simulink model "LocalPlannerMPCCascade"  (R2024b)
settings: Solver=FixedStepAuto  StartTime=0.0  StopTime=inf  FixedStep=0.1  RelTol=1e-3
StartFcn:
  | % clf
  | % rng(1,"twister");
  | % set_param([bdroot(gcb) '/TaskControllerIn/Simulink Signals/Confirm New Goal/newGoalBlock'],'Value','goalPose');
undefined symbols (not defined in the file or in its folder): fixedControllerParams, maxRefPathLen, nlobjTracking
settings Model: Creator=cstabile  LastModifiedBy=apattass
settings DataIOCC: SaveOutput=off  SaveTime=off
settings OptimizationCC: BlockReduction=off  EnhancedBackFolding=on  PassReuseOutputArgsAs=Individual arguments  ZeroExternalMemoryAtStartup=off  ZeroInternalMemoryAtStartup=off  MaxStackSize=64  OptimizeBlockOrder=speed  DifferentSizesBufferReuse=on  OptimizationCustomize=off  EfficientTunableParamExpr=on
settings DebuggingCC: IntegerOverflowMsg=none  ParameterTunabilityLossMsg=error
settings ModelReferenceCC: UpdateModelReferenceTargets=IfOutOfDate
settings SFSimCC: SFSimEcho=off  SimTargetLang=C++
settings RTWCC: Description=Embedded Coder  SystemTargetFile=ert.tlc  TemplateMakefile=ert_default_tmf  Toolchain=Colcon Tools  GPUComputeCapability=3.5
settings CodeAppCC: ForceParamTrailComments=on  IgnoreCustomStorageClasses=off  OperatorAnnotations=on  SimulinkDataObjDesc=on  SFDataObjDesc=on  InsertBlockDesc=on
settings ERTTargetCC: InlinedParameterPlacement=Hierarchical  RootIOFormat=Structure reference  ERTCustomFileTemplate=example_file_process.tlc  DynamicArrayContainerType=coder::array

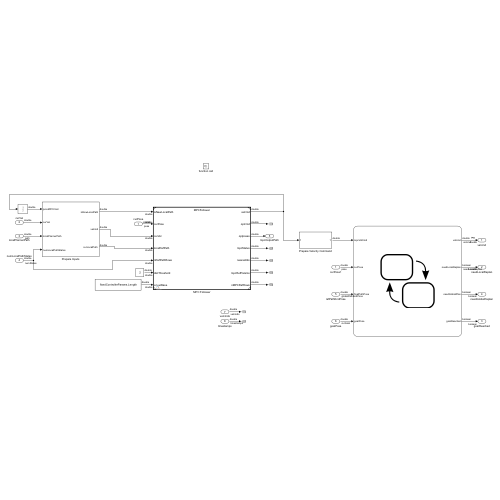
[thumbnail: Simulink's stored preview of the top-level diagram]
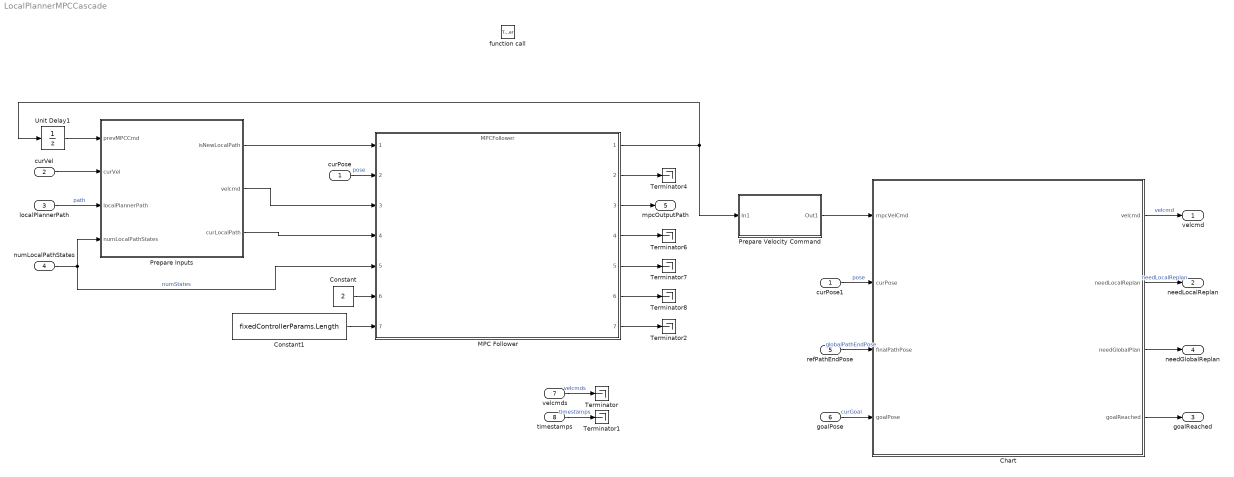
== system LocalPlannerMPCCascade ==
  curPose : Inport  OutDataTypeStr=double  PortDimensions=3  SampleTime=nlobjTracking.Ts
  curVel : Inport  Port=2  OutDataTypeStr=double  PortDimensions=[1 2]  SampleTime=nlobjTracking.Ts
  localPlannerPath : Inport  Port=3  OutDataTypeStr=double  PortDimensions=[1000 3]  SampleTime=nlobjTracking.Ts
  numLocalPathStates : Inport  Port=4  OutDataTypeStr=double  PortDimensions=1  SampleTime=nlobjTracking.Ts
  refPathEndPose : Inport  Port=5  OutDataTypeStr=double  PortDimensions=[1 3]
  goalPose : Inport  Port=6  OutDataTypeStr=double  PortDimensions=[1 3]
  velcmds : Inport  Port=7  OutDataTypeStr=double  PortDimensions=[1000 2]
  timestamps : Inport  Port=8  OutDataTypeStr=double  PortDimensions=[1000 1]
  function call : TriggerPort  TriggerType=function-call  VariantControl=(inherit)  SampleTimeType=periodic  SampleTime=nlobjTracking.Ts  PortDimensions=1  TriggerSignalSampleTime=[0.10000000000000001,0]
  Chart : Stateflow chart  TreatAsAtomicUnit=on
      settings: PortSchema="{\"entries\":[{\"content\":{\"sides\":[{\"content\":{\"connectorIds\":[\"In4\",\"In1\",\"In2\",\"In3\"]},\"type\":\"ConnectorPlacement.EquallySpacedRectSide\",\"uuid\":\"08395831-dbae-49cf-844d-729862efb56c\"},{\"content\":{\"connectorIds\":[\"Out4\",\"Out1\",\"Out2\",\"Out3\"],\"side\":\"RIGHT\"},\"type\":\"ConnectorPlacement.EquallySpacedRectSide\",\"uuid\":\"7aab2f4b-f147-41f5-84a6-1ccf26292ffc\"},{\"content\":{\"side\":\"TOP\"},\"type\":\"ConnectorPlacement.EquallySpacedRectSide\",\"uuid\":\"fd7335e6-a9e8-4ff2-a346-83748e189f04\"}]},\"type\":\"ConnectorPlacement.EquallySpacedConnector\",\"uuid\":\"68ab2c9d-d2a2-4341-98a3-3a3d7759d72e\"}],\"packageUris\":[\"http://schema.mathworks.com/mf0/Connector/R2020b\"],\"version\":\"1.0\"}"
  Constant : Constant  Value=2
  Constant1 : Constant  Value=fixedControllerParams.Length
  MPC Follower : ModelReference  ModelNameDialog=MPCFollower.slx  SimulationMode=Normal  ModelReferenceVersion=2.3
  Prepare Inputs : Subsystem
  Prepare Velocity Command : Subsystem
  Terminator{,1..2,4,6..8} (7 alike) : Terminator
  Unit Delay1 : UnitDelay  SampleTime=-1  HasFrameUpgradeWarning=on
  curPose1 : InportShadow  OutDataTypeStr=double  PortDimensions=3  SampleTime=nlobjTracking.Ts
  velcmd : Outport  OutDataTypeStr=double  PortDimensions=[1 2]
  needLocalReplan : Outport  Port=2  OutDataTypeStr=boolean  PortDimensions=1  OutputWhenDisabled=reset  InitialOutput=0
  goalReached : Outport  Port=3  OutDataTypeStr=boolean  PortDimensions=1  OutputWhenDisabled=reset  InitialOutput=0
  needGlobalReplan : Outport  Port=4  OutDataTypeStr=boolean  PortDimensions=1  OutputWhenDisabled=reset  InitialOutput=0
  mpcOutputPath : Outport  Port=5
  wires:
  Chart/2(needGlobalPlan) -> needGlobalReplan/1
  MPC Follower/2 -> Terminator4/1
  Chart/3(goalReached) -> goalReached/1
  Constant1/1 -> MPC Follower/7
  Constant/1 -> MPC Follower/6
  refPathEndPose/1 -> Chart/2(finalPathPose)  "globalPathEndPose"
  MPC Follower/6 -> Terminator8/1
  goalPose/1 -> Chart/3(goalPose)  "curGoal"
  MPC Follower/4 -> Terminator6/1
  MPC Follower/5 -> Terminator7/1
  velcmds/1 -> Terminator/1  "velcmds"
  timestamps/1 -> Terminator1/1  "timestamps"
  MPC Follower/7 -> Terminator2/1
  MPC Follower/1 -> Unit Delay1/1, Prepare Velocity Command/1(In1)
  Chart/4(velcmd) -> velcmd/1  "velcmd"
  Chart/1(needLocalReplan) -> needLocalReplan/1  "needLocalReplan"
  curPose/1 -> MPC Follower/2  "pose"
  curPose1/1 -> Chart/1(curPose)  "pose"
  Unit Delay1/1 -> Prepare Inputs/1(prevMPCCmd)
  localPlannerPath/1 -> Prepare Inputs/3(localPlannerPath)  "path"
  Prepare Inputs/1(isNewLocalPath) -> MPC Follower/1
  Prepare Inputs/2(velcmd) -> MPC Follower/3
  Prepare Inputs/3("curLocalPath ") -> MPC Follower/4
  numLocalPathStates/1 -> Prepare Inputs/4(numLocalPathStates), MPC Follower/5  "numStates"
  curVel/1 -> Prepare Inputs/2(curVel)
  Prepare Velocity Command/1(Out1) -> Chart/4(mpcVelCmd)
  MPC Follower/3 -> mpcOutputPath/1

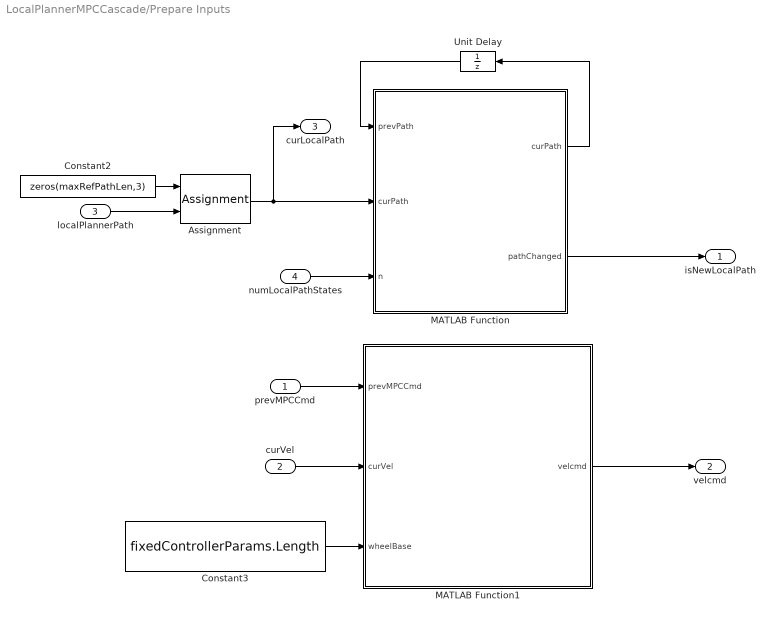
== system LocalPlannerMPCCascade/Prepare Inputs ==
  prevMPCCmd : Inport
  curVel : Inport  Port=2  SampleTime=nlobjTracking.Ts
  localPlannerPath : Inport  Port=3  SampleTime=nlobjTracking.Ts
  numLocalPathStates : Inport  Port=4  SampleTime=nlobjTracking.Ts
  Assignment : Assignment  NumberOfDimensions=2  DiagnosticForDimensions=Warning  IndexOptions=Starting index (dialog),Starting index (dialog)  Indices=1,1  OutputSizes=1,1
  Constant2 : Constant  Value=zeros(maxRefPathLen,3)
  Constant3 : Constant  Value=fixedControllerParams.Length
  MATLAB Function : MATLAB Function  TreatAsAtomicUnit=on
  MATLAB Function1 : MATLAB Function  TreatAsAtomicUnit=on
  Unit Delay : UnitDelay  SampleTime=-1  HasFrameUpgradeWarning=on
  isNewLocalPath : Outport
  velcmd : Outport  Port=2
  "curLocalPath " : Outport  Port=3
  wires:
  prevMPCCmd/1 -> MATLAB Function1/1(prevMPCCmd)
  MATLAB Function/2(pathChanged) -> isNewLocalPath/1
  MATLAB Function1/1(velcmd) -> velcmd/1
  curVel/1 -> MATLAB Function1/2(curVel)
  Assignment/1 -> "curLocalPath "/1, MATLAB Function/2("curPath ")
  Constant3/1 -> MATLAB Function1/3(wheelBase)
  Unit Delay/1 -> MATLAB Function/1(prevPath)
  Constant2/1 -> Assignment/1
  MATLAB Function/1(curPath) -> Unit Delay/1
  localPlannerPath/1 -> Assignment/2
  numLocalPathStates/1 -> MATLAB Function/3(n)

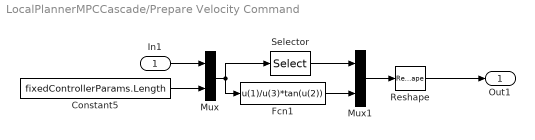
== system LocalPlannerMPCCascade/Prepare Velocity Command ==
  In1 : Inport
  Constant5 : Constant  Value=fixedControllerParams.Length
  Fcn1 : Fcn  Expr=u(1)/u(3)*tan(u(2))
  Mux : Mux  Inputs=2
  Mux1 : Mux  Inputs=2
  Reshape : Reshape  OutputDimensionality=Row vector (2-D)
  Selector : Selector  InputPortWidth=3  IndexOptions=Index vector (dialog)  Indices=1  OutputSizes=1
  Out1 : Outport
  wires:
  In1/1 -> Mux/1
  Mux/1 -> Fcn1/1, Selector/1
  Mux1/1 -> Reshape/1
  Fcn1/1 -> Mux1/2
  Reshape/1 -> Out1/1
  Constant5/1 -> Mux/2
  Selector/1 -> Mux1/1

== stateflow chart LocalPlannerMPCCascade/Chart ==
  (default) -> (junction 11) : {
      | needLocalReplan = false;
      | needGlobalPlan = false;
      | goalReached = false;
      | goalThreshold = 4.5;
      | }
  (junction 11) -> (junction 13) [order 1] : [poseReached(curPose,goalPose,goalThreshold,0.5)]
      | {goalReached = true;}
  (junction 11) -> (junction 15) [order 2]
  (junction 13) -> (junction 26)
  (junction 15) -> (junction 26) [order 1] : [poseReached(curPose,finalPathPose,goalThreshold,0)]
      | {needGlobalPlan = true;}
  (junction 26) -> (junction 30) : {velcmd = [0 0];}
  (junction 15) -> (junction 30) [order 2] : {velcmd = mpcVelCmd;}
  data: pose function_input; targetPose function_input; threshold function_input; orientationWeight function_input; isReached function_output; needLocalReplan output boolean; needGlobalPlan output boolean; curPose input; finalPathPose input; goalPose input; goalReached output boolean; velcmd output; goalThreshold local; mpcVelCmd input
  function isReached = poseReached(pose,targetPose,threshold,orientationWeight):
    | function isReached = poseReached(pose,targetPose,threshold,orientationWeight)
    |     arguments
    |         pose (1,3)
    |         targetPose (1,3)
    |         threshold (1,1) {mustBePositive} = 1;
    |         orientationWeight (1,1) {mustBeInRange(orientationWeight,0,1)} = 0;
    |     end
    |     dv = (pose-targetPose);
    |     dist = norm(dv.* [1 1 orientationWeight],2);
    |     isReached = dist <= threshold;
    | end

== matlab function LocalPlannerMPCCascade/Prepare Inputs/MATLAB Function ==
  data: prevPath input; curPath output; curPath input; pathChanged output; n input
function [curPath,pathChanged] = didPathChange(prevPath, curPath, n)
    pathChanged = double(~isequal(curPath(1:n,:),prevPath(1:n,:)));
end

== matlab function LocalPlannerMPCCascade/Prepare Inputs/MATLAB Function1 ==
  data: prevMPCCmd input; curVel input; velcmd output; wheelBase input
function velcmd = vel2mpc(prevMPCCmd,curVel,wheelBase)
velcmd = curVel;
if velcmd(1) == 0
    % Use previous steering angle when velocity is 0
    velcmd(2) = prevMPCCmd(2);
else
    % Otherwise compute it from turn-rate
    velcmd(2) = atan(curVel(2)*wheelBase/velcmd(1));
end
